simulink model "ex7_planar_robot_ct_PD_digi"  (R2016a)
settings: Solver=ode45  StartTime=0.0  StopTime=10  FixedStep=0.001  RelTol=1e-3
values from neighbouring files (symbols this model uses):
  a1 = u_gen(15)    [classical_joint_planar_robot_simulink.m]    (also in ct_gravit_planar_robot_simulink.m = u_gen(13); ct_pid_planar_robot_simulink.m; ct_planar_robot_simulink.m = u_gen(13); ex_planar_robot_2dof.m = 1)
  a2 = u_gen(16)    [classical_joint_planar_robot_simulink.m]    (also in ct_gravit_planar_robot_simulink.m = u_gen(14); ct_pid_planar_robot_simulink.m; ct_planar_robot_simulink.m = u_gen(14); ex_planar_robot_2dof.m = 1)
  g = u_gen(17)    [classical_joint_planar_robot_simulink.m]    (also in ct_gravit_planar_robot_simulink.m; ct_pid_planar_robot_simulink.m; ct_planar_robot_simulink.m = u_gen(15); ex_planar_robot_2dof.m = 9.81)
  m1 = u_gen(11)    [ac_controller_simulink.m]    (also in classical_joint_planar_robot_simulink.m = u_gen(13); ct_gravit_planar_robot_simulink.m; ct_pid_planar_robot_simulink.m = u_gen(13); ct_planar_robot_simulink.m)
  m2 = u_gen(12)    [ac_controller_simulink.m]    (also in classical_joint_planar_robot_simulink.m = u_gen(14); ct_gravit_planar_robot_simulink.m; ct_pid_planar_robot_simulink.m = u_gen(14); ct_planar_robot_simulink.m)
  Ts = 0.01    [ex_planar_robot_2dof.m]
settings Model: Creator=sevimeda  LastModifiedBy=sevimeda

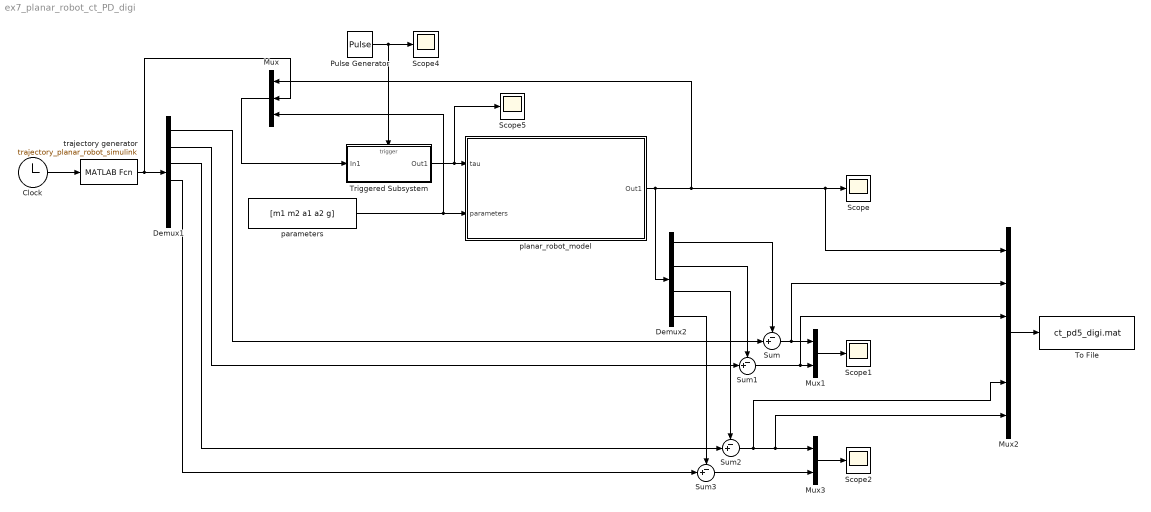
== system ex7_planar_robot_ct_PD_digi ==
  Clock : Clock
  Demux1 : Demux  Outputs=6
  Demux2 : Demux
  Mux : Mux  Inputs=3
  Mux1 : Mux  Inputs=2
  Mux2 : Mux  Inputs=6
  Mux3 : Mux  Inputs=2
  Pulse Generator : DiscretePulseGenerator  PulseType=Time based  Period=Ts  PulseWidth=50
  Scope{,1..2,4..5} (5 alike) : Scope
  Sum{,1..3} (4 alike) : Sum  Inputs=-+|
  To File : ToFile  Filename=ct_pd5_digi.mat  MatrixName=ct_pd
  Triggered Subsystem : Subsystem  TreatAsAtomicUnit=on
  parameters : Constant  Value=[m1 m2 a1 a2 g]
  planar_robot_model : Subsystem
  trajectory generator : MATLABFcn  MATLABFcn=trajectory_planar_robot_simulink
  wires:
  Clock/1 -> trajectory generator/1
  trajectory generator/1 -> Demux1/1, Mux/2
  parameters/1 -> planar_robot_model/2(parameters), Mux/3
  planar_robot_model/1(Out1) -> Mux/1, Mux2/1, Scope/1, Demux2/1
  Demux1/1 -> Sum/2
  Demux2/1 -> Sum/1
  Sum/1 -> Mux1/1, Mux2/2
  Demux2/2 -> Sum1/1
  Sum1/1 -> Mux2/3, Mux1/2
  Demux1/2 -> Sum1/2
  Sum2/1 -> Mux2/5, Mux2/6, Mux3/1
  Sum3/1 -> Mux3/2
  Demux2/3 -> Sum2/1
  Demux2/4 -> Sum3/1
  Demux1/3 -> Sum2/2
  Demux1/4 -> Sum3/2
  Mux1/1 -> Scope1/1
  Mux3/1 -> Scope2/1
  Mux2/1 -> To File/1
  Mux/1 -> Triggered Subsystem/1(In1)
  Triggered Subsystem/1(Out1) -> Scope5/1, planar_robot_model/1(tau)
  Pulse Generator/1 -> Scope4/1, Triggered Subsystem/Trigger

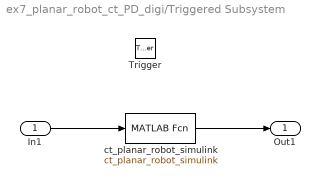
== system ex7_planar_robot_ct_PD_digi/Triggered Subsystem ==
  In1 : Inport
  Trigger : TriggerPort  VariantControl=Variant
  ct_planar_robot_simulink : MATLABFcn  MATLABFcn=ct_planar_robot_simulink
  Out1 : Outport
  wires:
  In1/1 -> ct_planar_robot_simulink/1
  ct_planar_robot_simulink/1 -> Out1/1

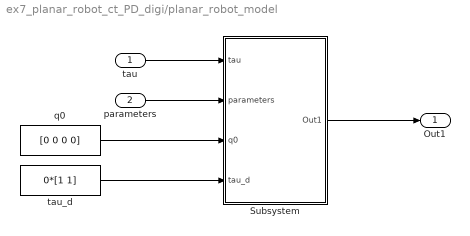
== system ex7_planar_robot_ct_PD_digi/planar_robot_model ==
  tau : Inport
  parameters : Inport  Port=2
  Subsystem : Subsystem
  q0 : Constant  Value=[0 0 0 0]
  tau_d : Constant  Value=0*[1 1]
  Out1 : Outport
  wires:
  Subsystem/1(Out1) -> Out1/1
  q0/1 -> Subsystem/3(q0)
  tau_d/1 -> Subsystem/4(tau_d)
  tau/1 -> Subsystem/1(tau)
  parameters/1 -> Subsystem/2(parameters)

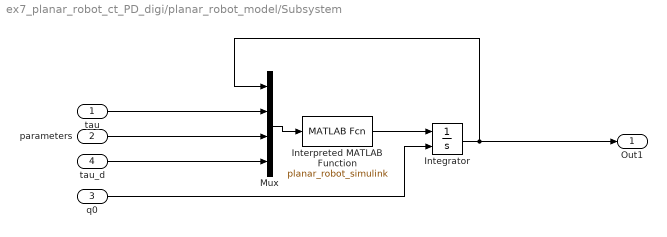
== system ex7_planar_robot_ct_PD_digi/planar_robot_model/Subsystem ==
  tau : Inport
  parameters : Inport  Port=2
  q0 : Inport  Port=3
  tau_d : Inport  Port=4
  Integrator : Integrator  InitialConditionSource=external
  Interpreted MATLAB Function : MATLABFcn  MATLABFcn=planar_robot_simulink  OutputDimensions=4
  Mux : Mux
  Out1 : Outport
  wires:
  Interpreted MATLAB Function/1 -> Integrator/1
  q0/1 -> Integrator/2
  Mux/1 -> Interpreted MATLAB Function/1
  Integrator/1 -> Out1/1, Mux/1
  tau/1 -> Mux/2
  parameters/1 -> Mux/3
  tau_d/1 -> Mux/4
